simulink library "AsdRouterBtc"  (R2022b)
settings: Solver=VariableStepAuto  StartTime=0.0  StopTime=10.0  RelTol=1e-3
libraries: RTC x5, TuneVar x2, FeaturePath x1, HandyTextFile x1, dspindex x1
settings Model: Creator=kl13806  LastModifiedBy=kl13806
settings SolverCC: AlgebraicLoopSolver=TrustRegion
settings DebuggingCC: UnconnectedInputMsg=warning  UnconnectedOutputMsg=warning  UnconnectedLineMsg=warning  SFMachineParentedDataDiag=warning
settings ModelReferenceCC: EnableRefExpFcnMdlSchedulingChecks=on
settings RTWCC: DLArmComputeVersion=19.05

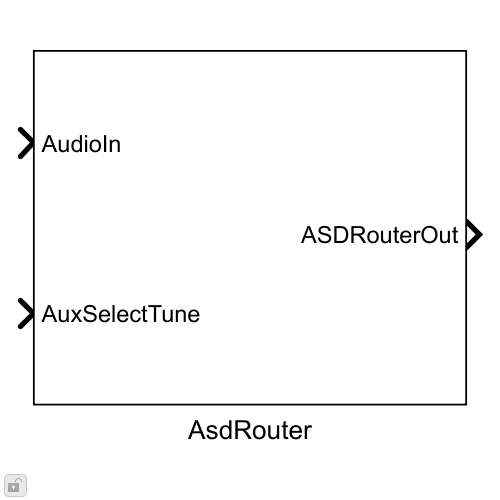
[thumbnail: Simulink's stored preview of the top-level diagram]
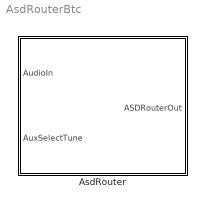
== system AsdRouterBtc ==
  AsdRouter : Subsystem  mask(Blocklib AsdRouter){Config=[], FeatureName=ASDRouter}
      mask prompts: Config "AsdRouterConfig"; FeatureName "Feature path name:"
      mask init:
      | blkh=gcbh;
      | Config=BTConfig.Assert(blkh,Config);
      | Config.Validate();
      | BTConfig.InitSetFeatureIfPresent(blkh,'FeatureName');
      | 
      | % Most significant bit (MSB) of RTC parameters is used to switch between RTC
      | % & TuneTOP configurations. If MSB of any RTC parameter is set to '1' means
      | % TuneTOP values will be used. By default TuneTOP configurations are to be used, so MSB of all RTC parameters
      | % is set to '1' by initializing with negative number.
      | mainSelectRTCInit = -ones(1,Config.NumChanOut);
      | enableAuxRTCInit = -ones(1,length(Config.NumAux));
      | auxSelectRTCInit = -ones(1,Config.NumChanOut*length(Config.NumAux));
      mask Callback Config: BTConfig.CallbackHideIfPresent(gcbh,{'FeatureName'});
      mask TypeOptions FeatureName: FeaturePath/FeatureName

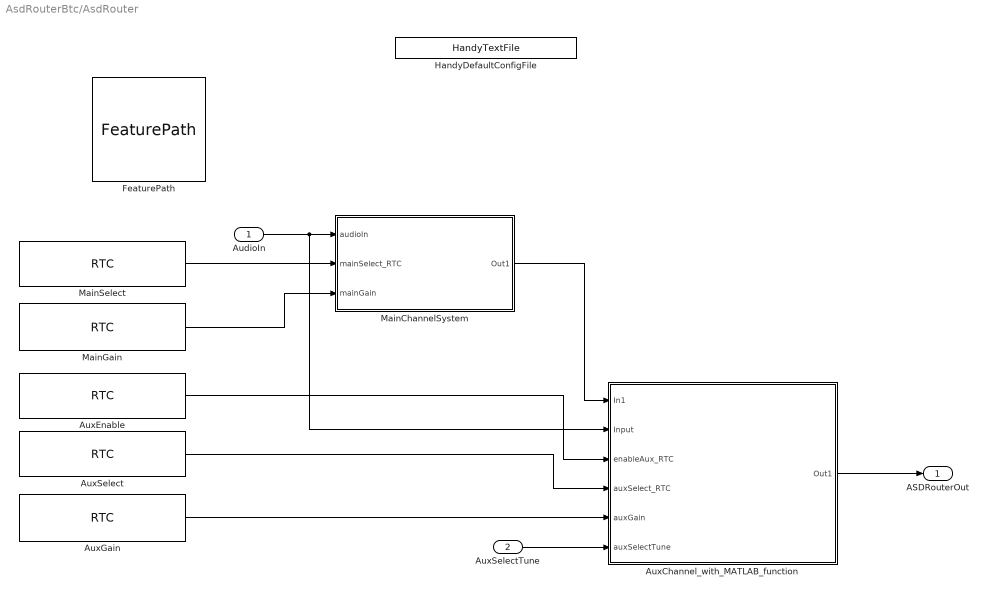
== system AsdRouterBtc/AsdRouter ==
  AudioIn : Inport
  AuxSelectTune : Inport  Port=2
  AuxChannel_with_MATLAB_function : Subsystem
  AuxEnable : RTC/RTC  REQ_Priority=RTC_Mask.NormalPriority  RequestAtInit=off  EnableRequest=off  REQElemName1=EnableAuxFlag  REQElemType1=int32  REQElemWidth1=length(Config.NumAux)  REQElemInitial1=enableAuxRTCInit  REQElemType2=single  REQElemWidth2=1  REQElemInitial2=[]  REQElemType3=int8  REQElemWidth3=1  REQElemInitial3=[]  REQElemType4=int8  REQElemWidth4=1  REQElemInitial4=[]  REQElemType5=single  REQElemWidth5=1  REQElemInitial5=[]  REQElemType6=uint32  REQElemWidth6=1  REQElemInitial6=[]  REQElemType7=uint32  REQElemWidth7=1  REQElemInitial7=[]  REQElemType8=uint32  REQElemWidth8=1  REQElemInitial8=[]  REQElemType9=uint32  REQElemWidth9=1  REQElemInitial9=[]  REQElemType10=uint32  REQElemWidth10=1  REQElemInitial10=[]  EnableResponse=on  EnableRSP_StatusIn=off  RSPElemType1=uint32  RSPElemWidth1=1  RSPElemType2=uint32  RSPElemWidth2=1  RSPElemType3=uint32  RSPElemWidth3=1  RSPElemType4=uint32  RSPElemWidth4=1  RSPElemType5=uint32  RSPElemWidth5=1  RSPElemType6=uint32  RSPElemWidth6=1  RSPElemType7=uint32  RSPElemWidth7=1  RSPElemType8=uint32  RSPElemWidth8=1  RSPElemType9=uint32  RSPElemWidth9=1  RSPElemType10=uint32  RSPElemWidth10=1  EnableNotification=off  EnableNTF_PrepTrig=off  NTFElemType1=uint32  NTFElemWidth1=1  NTFElemType2=uint32  NTFElemWidth2=1  NTFElemType3=uint32  NTFElemWidth3=1  NTFElemType4=uint32  NTFElemWidth4=1  NTFElemType5=uint32  NTFElemWidth5=1  NTFElemType6=uint32  NTFElemWidth6=1  NTFElemType7=uint32  NTFElemWidth7=1  NTFElemType8=uint32  NTFElemWidth8=1  NTFElemType9=uint32  NTFElemWidth9=1  NTFElemType10=uint32  NTFElemWidth10=1  MaskMessageName=AuxEnable
      settings: SourceProductName=Bose Talaria
  AuxGain : RTC/RTC  REQ_Priority=RTC_Mask.NormalPriority  RequestAtInit=off  EnableRequest=off  REQElemName1=AuxGain  REQElemType1=single  REQElemWidth1=Config.NumChanOut*length(Config.NumAux)  REQElemInitial1=Config.AuxGain  REQElemType2=single  REQElemWidth2=1  REQElemInitial2=[]  REQElemType3=int8  REQElemWidth3=1  REQElemInitial3=[]  REQElemType4=int8  REQElemWidth4=1  REQElemInitial4=[]  REQElemType5=single  REQElemWidth5=1  REQElemInitial5=[]  REQElemType6=uint32  REQElemWidth6=1  REQElemInitial6=[]  REQElemType7=uint32  REQElemWidth7=1  REQElemInitial7=[]  REQElemType8=uint32  REQElemWidth8=1  REQElemInitial8=[]  REQElemType9=uint32  REQElemWidth9=1  REQElemInitial9=[]  REQElemType10=uint32  REQElemWidth10=1  REQElemInitial10=[]  EnableResponse=on  EnableRSP_StatusIn=off  RSPElemType1=uint32  RSPElemWidth1=1  RSPElemType2=uint32  RSPElemWidth2=1  RSPElemType3=uint32  RSPElemWidth3=1  RSPElemType4=uint32  RSPElemWidth4=1  RSPElemType5=uint32  RSPElemWidth5=1  RSPElemType6=uint32  RSPElemWidth6=1  RSPElemType7=uint32  RSPElemWidth7=1  RSPElemType8=uint32  RSPElemWidth8=1  RSPElemType9=uint32  RSPElemWidth9=1  RSPElemType10=uint32  RSPElemWidth10=1  EnableNotification=off  EnableNTF_PrepTrig=off  NTFElemType1=uint32  NTFElemWidth1=1  NTFElemType2=uint32  NTFElemWidth2=1  NTFElemType3=uint32  NTFElemWidth3=1  NTFElemType4=uint32  NTFElemWidth4=1  NTFElemType5=uint32  NTFElemWidth5=1  NTFElemType6=uint32  NTFElemWidth6=1  NTFElemType7=uint32  NTFElemWidth7=1  NTFElemType8=uint32  NTFElemWidth8=1  NTFElemType9=uint32  NTFElemWidth9=1  NTFElemType10=uint32  NTFElemWidth10=1  MaskMessageName=AuxGain
      settings: SourceProductName=Bose Talaria
  AuxSelect : RTC/RTC  REQ_Priority=RTC_Mask.NormalPriority  RequestAtInit=off  EnableRequest=off  REQElemName1=AuxSelect  REQElemType1=int32  REQElemWidth1=Config.NumChanOut*length(Config.NumAux)  REQElemInitial1=auxSelectRTCInit  REQElemType2=single  REQElemWidth2=1  REQElemInitial2=[]  REQElemType3=int8  REQElemWidth3=1  REQElemInitial3=[]  REQElemType4=int8  REQElemWidth4=1  REQElemInitial4=[]  REQElemType5=single  REQElemWidth5=1  REQElemInitial5=[]  REQElemType6=uint32  REQElemWidth6=1  REQElemInitial6=[]  REQElemType7=uint32  REQElemWidth7=1  REQElemInitial7=[]  REQElemType8=uint32  REQElemWidth8=1  REQElemInitial8=[]  REQElemType9=uint32  REQElemWidth9=1  REQElemInitial9=[]  REQElemType10=uint32  REQElemWidth10=1  REQElemInitial10=[]  EnableResponse=on  EnableRSP_StatusIn=off  RSPElemType1=uint32  RSPElemWidth1=1  RSPElemType2=uint32  RSPElemWidth2=1  RSPElemType3=uint32  RSPElemWidth3=1  RSPElemType4=uint32  RSPElemWidth4=1  RSPElemType5=uint32  RSPElemWidth5=1  RSPElemType6=uint32  RSPElemWidth6=1  RSPElemType7=uint32  RSPElemWidth7=1  RSPElemType8=uint32  RSPElemWidth8=1  RSPElemType9=uint32  RSPElemWidth9=1  RSPElemType10=uint32  RSPElemWidth10=1  EnableNotification=off  EnableNTF_PrepTrig=off  NTFElemType1=uint32  NTFElemWidth1=1  NTFElemType2=uint32  NTFElemWidth2=1  NTFElemType3=uint32  NTFElemWidth3=1  NTFElemType4=uint32  NTFElemWidth4=1  NTFElemType5=uint32  NTFElemWidth5=1  NTFElemType6=uint32  NTFElemWidth6=1  NTFElemType7=uint32  NTFElemWidth7=1  NTFElemType8=uint32  NTFElemWidth8=1  NTFElemType9=uint32  NTFElemWidth9=1  NTFElemType10=uint32  NTFElemWidth10=1  MaskMessageName=AuxSelect
      settings: SourceProductName=Bose Talaria
  FeaturePath : FeaturePath/FeaturePath  FeatureName=ASDRouter  IsGroup=off  GroupNumber=-1  IsModule=off  TriggerInit=[-50 -126 65 -19]
      settings: SourceProductName=Bose Talaria
  HandyDefaultConfigFile : HandyTextFile/HandyTextFile  TemplateSource=Config  FileSuffix=Init  OpenDialogOnLoad=off  UseThisBlockName=off  AddGrandParentNamePrefix=off  TheDefaultText=|  ShowInLibBrowser=on
      | % $(FILENAME) Setup model parameters for each "Init" callback (e.g. update diagram)
      | sample_rate_in_hertz = 44100;
      | frame_size = 32;
      | sysin_channel_count = 2;
      settings: SourceProductName=Bose Talaria
  MainChannelSystem : Subsystem
  MainGain : RTC/RTC  REQ_Priority=RTC_Mask.NormalPriority  RequestAtInit=off  EnableRequest=off  REQElemName1=mainGain  REQElemType1=single  REQElemWidth1=Config.NumChanOut  REQElemInitial1=Config.MainGain  REQElemType2=single  REQElemWidth2=1  REQElemInitial2=[]  REQElemType3=int8  REQElemWidth3=1  REQElemInitial3=[]  REQElemType4=int8  REQElemWidth4=1  REQElemInitial4=[]  REQElemType5=single  REQElemWidth5=1  REQElemInitial5=[]  REQElemType6=uint32  REQElemWidth6=1  REQElemInitial6=[]  REQElemType7=uint32  REQElemWidth7=1  REQElemInitial7=[]  REQElemType8=uint32  REQElemWidth8=1  REQElemInitial8=[]  REQElemType9=uint32  REQElemWidth9=1  REQElemInitial9=[]  REQElemType10=uint32  REQElemWidth10=1  REQElemInitial10=[]  EnableResponse=on  EnableRSP_StatusIn=off  RSPElemType1=uint32  RSPElemWidth1=1  RSPElemType2=uint32  RSPElemWidth2=1  RSPElemType3=uint32  RSPElemWidth3=1  RSPElemType4=uint32  RSPElemWidth4=1  RSPElemType5=uint32  RSPElemWidth5=1  RSPElemType6=uint32  RSPElemWidth6=1  RSPElemType7=uint32  RSPElemWidth7=1  RSPElemType8=uint32  RSPElemWidth8=1  RSPElemType9=uint32  RSPElemWidth9=1  RSPElemType10=uint32  RSPElemWidth10=1  EnableNotification=off  EnableNTF_PrepTrig=off  NTFElemType1=uint32  NTFElemWidth1=1  NTFElemType2=uint32  NTFElemWidth2=1  NTFElemType3=uint32  NTFElemWidth3=1  NTFElemType4=uint32  NTFElemWidth4=1  NTFElemType5=uint32  NTFElemWidth5=1  NTFElemType6=uint32  NTFElemWidth6=1  NTFElemType7=uint32  NTFElemWidth7=1  NTFElemType8=uint32  NTFElemWidth8=1  NTFElemType9=uint32  NTFElemWidth9=1  NTFElemType10=uint32  NTFElemWidth10=1  MaskMessageName=MainGain
      settings: SourceProductName=Bose Talaria
  MainSelect : RTC/RTC  REQ_Priority=RTC_Mask.NormalPriority  RequestAtInit=off  EnableRequest=off  REQElemName1=mainSelect  REQElemType1=int32  REQElemWidth1=Config.NumChanOut  REQElemInitial1=mainSelectRTCInit  REQElemType2=single  REQElemWidth2=1  REQElemInitial2=[]  REQElemType3=int8  REQElemWidth3=1  REQElemInitial3=[]  REQElemType4=int8  REQElemWidth4=1  REQElemInitial4=[]  REQElemType5=single  REQElemWidth5=1  REQElemInitial5=[]  REQElemType6=uint32  REQElemWidth6=1  REQElemInitial6=[]  REQElemType7=uint32  REQElemWidth7=1  REQElemInitial7=[]  REQElemType8=uint32  REQElemWidth8=1  REQElemInitial8=[]  REQElemType9=uint32  REQElemWidth9=1  REQElemInitial9=[]  REQElemType10=uint32  REQElemWidth10=1  REQElemInitial10=[]  EnableResponse=on  EnableRSP_StatusIn=off  RSPElemType1=uint32  RSPElemWidth1=1  RSPElemType2=uint32  RSPElemWidth2=1  RSPElemType3=uint32  RSPElemWidth3=1  RSPElemType4=uint32  RSPElemWidth4=1  RSPElemType5=uint32  RSPElemWidth5=1  RSPElemType6=uint32  RSPElemWidth6=1  RSPElemType7=uint32  RSPElemWidth7=1  RSPElemType8=uint32  RSPElemWidth8=1  RSPElemType9=uint32  RSPElemWidth9=1  RSPElemType10=uint32  RSPElemWidth10=1  EnableNotification=off  EnableNTF_PrepTrig=off  NTFElemType1=uint32  NTFElemWidth1=1  NTFElemType2=uint32  NTFElemWidth2=1  NTFElemType3=uint32  NTFElemWidth3=1  NTFElemType4=uint32  NTFElemWidth4=1  NTFElemType5=uint32  NTFElemWidth5=1  NTFElemType6=uint32  NTFElemWidth6=1  NTFElemType7=uint32  NTFElemWidth7=1  NTFElemType8=uint32  NTFElemWidth8=1  NTFElemType9=uint32  NTFElemWidth9=1  NTFElemType10=uint32  NTFElemWidth10=1  MaskMessageName=MainSelect
      settings: SourceProductName=Bose Talaria
  ASDRouterOut : Outport  VectorParamsAs1DForOutWhenUnconnected=off
  wires:
  AudioIn/1 -> AuxChannel_with_MATLAB_function/2(Input), MainChannelSystem/1(audioIn)
  AuxChannel_with_MATLAB_function/1(Out1) -> ASDRouterOut/1
  MainChannelSystem/1(Out1) -> AuxChannel_with_MATLAB_function/1(In1)
  MainGain/1 -> MainChannelSystem/3(mainGain)
  AuxGain/1 -> AuxChannel_with_MATLAB_function/5(auxGain)
  AuxSelect/1 -> AuxChannel_with_MATLAB_function/4(auxSelect_RTC)
  AuxEnable/1 -> AuxChannel_with_MATLAB_function/3(enableAux_RTC)
  MainSelect/1 -> MainChannelSystem/2(mainSelect_RTC)
  AuxSelectTune/1 -> AuxChannel_with_MATLAB_function/6(auxSelectTune)

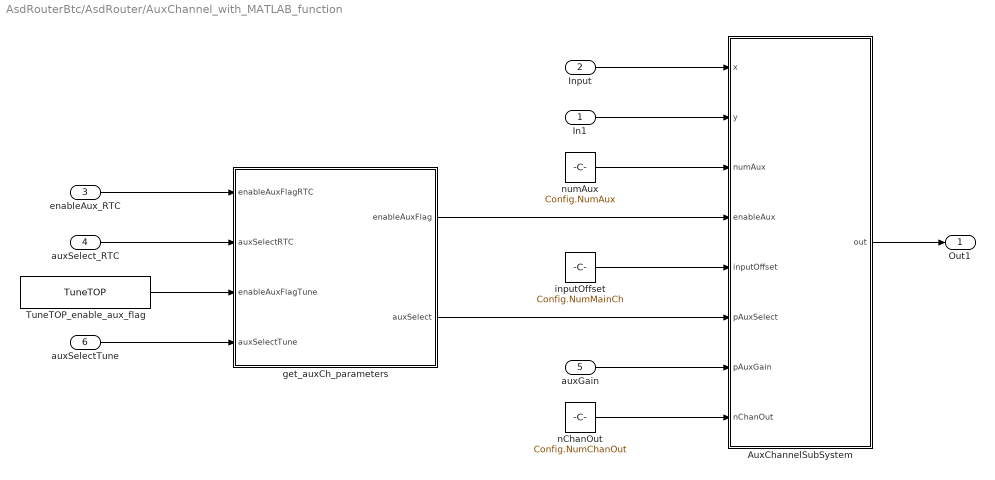
== system AsdRouterBtc/AsdRouter/AuxChannel_with_MATLAB_function ==
  In1 : Inport  PortDimensions=[Config.FrameSize Config.NumChanOut]
  Input : Inport  Port=2
  enableAux_RTC : Inport  Port=3
  auxSelect_RTC : Inport  Port=4
  auxGain : Inport  Port=5
  auxSelectTune : Inport  Port=6
  AuxChannelSubSystem : MATLAB Function  TreatAsAtomicUnit=on
  TuneTOP_enable_aux_flag : TuneVar/TuneTOP  TriggerInit=[-445 144 -315 176]  TopName=EnableAux  TuneName=EnableAux  DataType=int32  TunabilityNumber=1  MinValue=[]  MaxValue=[]  BankNumber=0  PreOverlay=false  PostOverlay=false  UseSameName=on  MaskValue=Config.EnableAux
      settings: SourceProductName=Bose Talaria
  get_auxCh_parameters : MATLAB Function  TreatAsAtomicUnit=on
  inputOffset : Constant  Value=Config.NumMainCh  OutDataTypeStr=int32
  nChanOut : Constant  Value=Config.NumChanOut  OutDataTypeStr=int32
  numAux : Constant  Value=Config.NumAux  OutDataTypeStr=int32
  Out1 : Outport  PortDimensions=[Config.FrameSize Config.NumChanOut]  VectorParamsAs1DForOutWhenUnconnected=off
  wires:
  In1/1 -> AuxChannelSubSystem/2(y)
  AuxChannelSubSystem/1(out) -> Out1/1
  Input/1 -> AuxChannelSubSystem/1(x)
  numAux/1 -> AuxChannelSubSystem/3(numAux)
  TuneTOP_enable_aux_flag/1 -> get_auxCh_parameters/3(enableAuxFlagTune)
  inputOffset/1 -> AuxChannelSubSystem/5(inputOffset)
  nChanOut/1 -> AuxChannelSubSystem/8(nChanOut)
  auxSelectTune/1 -> get_auxCh_parameters/4(auxSelectTune)
  auxGain/1 -> AuxChannelSubSystem/7(pAuxGain)
  enableAux_RTC/1 -> get_auxCh_parameters/1(enableAuxFlagRTC)
  auxSelect_RTC/1 -> get_auxCh_parameters/2(auxSelectRTC)
  get_auxCh_parameters/1(enableAuxFlag) -> AuxChannelSubSystem/4(enableAux)
  get_auxCh_parameters/2(auxSelect) -> AuxChannelSubSystem/6(pAuxSelect)

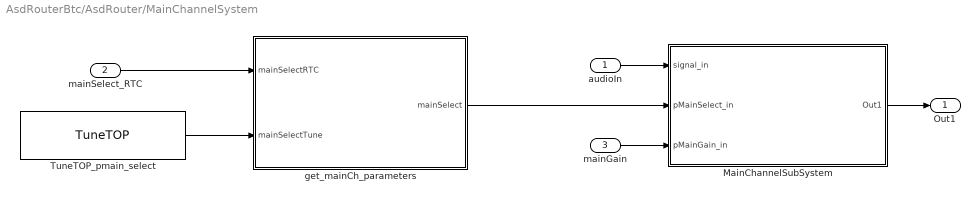
== system AsdRouterBtc/AsdRouter/MainChannelSystem ==
  audioIn : Inport
  mainSelect_RTC : Inport  Port=2
  mainGain : Inport  Port=3
  MainChannelSubSystem : Subsystem  TreatAsAtomicUnit=on
  TuneTOP_pmain_select : TuneVar/TuneTOP  TriggerInit=[-390 156 -225 204]  TopName=MainSelect  TuneName=MainSelect  DataType=int32  TunabilityNumber=1  MinValue=[]  MaxValue=[]  BankNumber=0  PreOverlay=false  PostOverlay=false  UseSameName=on  MaskValue=Config.MainSelect
      settings: SourceProductName=Bose Talaria
  get_mainCh_parameters : MATLAB Function  TreatAsAtomicUnit=on
  Out1 : Outport  PortDimensions=[Config.FrameSize Config.NumChanOut]  VectorParamsAs1DForOutWhenUnconnected=off
  wires:
  MainChannelSubSystem/1(Out1) -> Out1/1
  audioIn/1 -> MainChannelSubSystem/1(signal_in)
  TuneTOP_pmain_select/1 -> get_mainCh_parameters/2(mainSelectTune)
  mainGain/1 -> MainChannelSubSystem/3(pMainGain_in)
  get_mainCh_parameters/1(mainSelect) -> MainChannelSubSystem/2(pMainSelect_in)
  mainSelect_RTC/1 -> get_mainCh_parameters/1(mainSelectRTC)

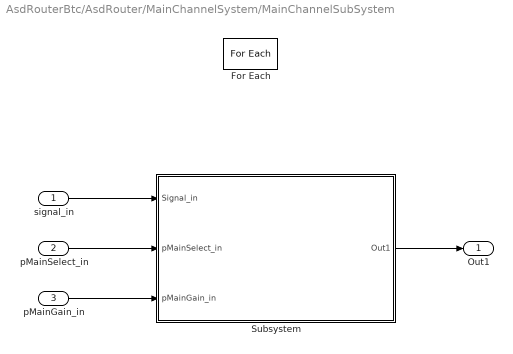
== system AsdRouterBtc/AsdRouter/MainChannelSystem/MainChannelSubSystem ==
  signal_in : Inport
  pMainSelect_in : Inport  Port=2  Partition=on  PartitionDimension=1  PartitionWidth=1  PartitionOffset=0
  pMainGain_in : Inport  Port=3  Partition=on  PartitionDimension=1  PartitionWidth=1  PartitionOffset=0
  For Each : ForEach  DisableCoverage=on
  Subsystem : Subsystem
  Out1 : Outport  ConcatenationDimension=2  VectorParamsAs1DForOutWhenUnconnected=off
  wires:
  Subsystem/1(Out1) -> Out1/1
  signal_in/1 -> Subsystem/1(Signal_in)
  pMainSelect_in/1 -> Subsystem/2(pMainSelect_in)
  pMainGain_in/1 -> Subsystem/3(pMainGain_in)

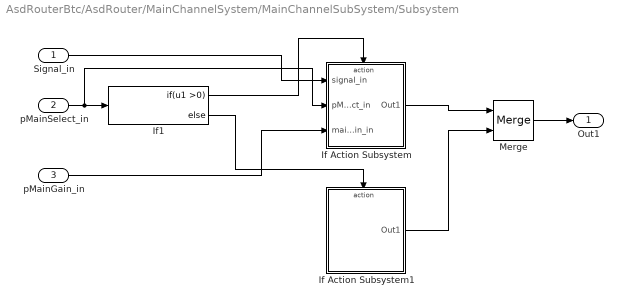
== system AsdRouterBtc/AsdRouter/MainChannelSystem/MainChannelSubSystem/Subsystem ==
  Signal_in : Inport
  pMainSelect_in : Inport  Port=2
  pMainGain_in : Inport  Port=3
  If Action Subsystem : Subsystem  TreatAsAtomicUnit=on
  If Action Subsystem1 : Subsystem  TreatAsAtomicUnit=on
  If1 : If  IfExpression=u1 >0
  Merge : Merge
  Out1 : Outport  VectorParamsAs1DForOutWhenUnconnected=off
  wires:
  pMainSelect_in/1 -> If Action Subsystem/2(pMainSelect_in), If1/1
  If1/1 -> If Action Subsystem/Action
  Signal_in/1 -> If Action Subsystem/1(signal_in)
  pMainGain_in/1 -> If Action Subsystem/3(mainGain_in)
  If Action Subsystem/1(Out1) -> Merge/1
  If Action Subsystem1/1(Out1) -> Merge/2
  Merge/1 -> Out1/1
  If1/2 -> If Action Subsystem1/Action

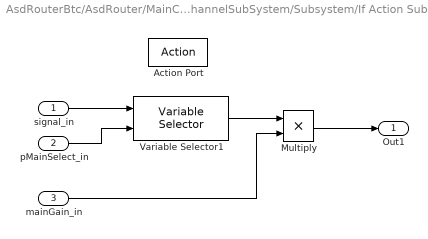
== system AsdRouterBtc/AsdRouter/MainChannelSystem/MainChannelSubSystem/Subsystem/If Action Subsystem ==
  signal_in : Inport
  pMainSelect_in : Inport  Port=2
  mainGain_in : Inport  Port=3
  Action Port : ActionPort
  Multiply : Product
  Variable Selector1 : dspindex/Variable Selector  NumInputs=1  rowsOrCols=Columns  IdxMode=Variable  Elements=tempSelect  ZerOneIdxMode=One-based  errmode=Clip Index  FillMode=on  FillValues=0
  Out1 : Outport  VectorParamsAs1DForOutWhenUnconnected=off
  wires:
  mainGain_in/1 -> Multiply/2
  Multiply/1 -> Out1/1
  Variable Selector1/1 -> Multiply/1
  signal_in/1 -> Variable Selector1/1
  pMainSelect_in/1 -> Variable Selector1/2

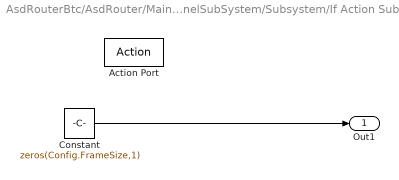
== system AsdRouterBtc/AsdRouter/MainChannelSystem/MainChannelSubSystem/Subsystem/If Action Subsystem1 ==
  Action Port : ActionPort
  Constant : Constant  Value=zeros(Config.FrameSize,1)  OutDataTypeStr=single
  Out1 : Outport  VectorParamsAs1DForOutWhenUnconnected=off
  wires:
  Constant/1 -> Out1/1

== matlab function AsdRouterBtc/AsdRouter/MainChannelSystem/get_mainCh_parameters ==
  data: mainSelectRTC input; mainSelect output; mainSelectTune input
function mainSelect  = get_mainChannel_parameters(mainSelectRTC,... % RTC message parameter
                        mainSelectTune) % Tune parameter

% Main Select is provided to the block through Tune variables. However 
% if parameters are provided through RTC, the block will use the values 
% given in the RTC messages.    
mainSelect = int32(mainSelectTune);
for ind=1:size(mainSelectRTC,1)
% If MSB of mainSelectRTC is set to '1', it means Tune values are to be used and not RTC value
    if (~bitget(mainSelectRTC(ind),32))
        mainSelect(ind) = mainSelectRTC(ind);        
    end
end

== matlab function AsdRouterBtc/AsdRouter/AuxChannel_with_MATLAB_function/AuxChannelSubSystem ==
  data: x input; out output; y input; numAux input; enableAux input; inputOffset input; pAuxSelect input; pAuxGain input; nChanOut input
function out = fcn(x, y, numAux, enableAux, inputOffset, pAuxSelect, pAuxGain, nChanOut)
% initial inputOffset is the number of ENT inputs

for i=1:length(numAux)
    if(enableAux(i))
        tempSelect = inputOffset + pAuxSelect((i-1)*nChanOut+1:i*nChanOut);   % Account for Matlab 1 index
        tempGain = pAuxGain((i-1)*nChanOut+1:i*nChanOut);   % Account for Matlab 1 index
        for ch = 1:1:nChanOut
            if (tempSelect(ch) > inputOffset)
                % This channel is part of AUX, not MAIN
                if(tempSelect(ch) > (numAux(i)+inputOffset))
                    % aux select index exceeds number of aux inputs of that bank
                    y(:,ch)=y(:,ch) + x(:, tempSelect(ch)) * 0;
                else
                    y(:,ch)=y(:,ch) + x(:, tempSelect(ch)) * tempGain(ch);
                end
            end
        end
    end
    inputOffset = inputOffset + numAux(i);
end
out = y;

== matlab function AsdRouterBtc/AsdRouter/AuxChannel_with_MATLAB_function/get_auxCh_parameters ==
  data: enableAuxFlag output; enableAuxFlagRTC input; auxSelectRTC input; auxSelect output; enableAuxFlagTune input; auxSelectTune input
function [enableAuxFlag, auxSelect] = get_auxChannel_parameters(...
    enableAuxFlagRTC, auxSelectRTC,... % RTC message parameters
    enableAuxFlagTune, auxSelectTune) % Tune parameters

% Aux Select and Enable Aux are provided to the block through Tune variables. However 
% if parameters are provided through RTC, the block will use the values 
% given in the RTC messages.    
enableAuxFlag = int32(enableAuxFlagTune);
auxSelect = int32(auxSelectTune);

% If MSB of auxSelectRTC/enableAuxFlagRTC is set to '1', it means Tune
% values are to be used and not RTC values
for ind=1:size(auxSelectRTC,1)
    if (~bitget(auxSelectRTC(ind),32))
        auxSelect(ind) = auxSelectRTC(ind);                
    end
end

for ind=1:length(enableAuxFlagRTC)
    if(~bitget(enableAuxFlagRTC(ind),32))
        enableAuxFlag(ind) = enableAuxFlagRTC(ind);
    end
end
